simulink model "circuitElectrique"  (R2014b)
settings: Solver=ode23tb  StartTime=t0  StopTime=tf  MaxStep=max_step  MinStep=min_step  RelTol=tol
StopFcn:
  | save(wSaveFileName,wLinearOutputName,wNonLinearOutputName)
values from neighbouring files (symbols this model uses):
  A = [-3/(8*Ca)*Ei_mean^2-1/(R*Ca), 1/Ca;-1/L,0]    [circuitElectriqueDataDictionnary (Copie en conflit de Adam Burney 2015-02-07).m]    (also in circuitElectriqueDataDictionnary.m)
  Ai = Ais(i)    [circuitElectriqueDataDictionnary (Copie en conflit de Adam Burney 2015-02-07).m]    (also in circuitElectriqueDataDictionnary.m)
  alpha = 3    [circuitElectriqueDataDictionnary (Copie en conflit de Adam Burney 2015-02-07).m]    (also in circuitElectriqueDataDictionnary.m)
  B = [1/(R*Ca);1/L]    [circuitElectriqueDataDictionnary (Copie en conflit de Adam Burney 2015-02-07).m]    (also in circuitElectriqueDataDictionnary.m)
  C = eye(2)    [circuitElectriqueDataDictionnary (Copie en conflit de Adam Burney 2015-02-07).m]    (also in circuitElectriqueDataDictionnary.m)
  D = [0;0]    [circuitElectriqueDataDictionnary (Copie en conflit de Adam Burney 2015-02-07).m]    (also in circuitElectriqueDataDictionnary.m)
  Ei = 2    [circuitElectriqueDataDictionnary (Copie en conflit de Adam Burney 2015-02-07).m]    (also in circuitElectriqueDataDictionnary.m)
  Io = 1/8    (= 0.125)    [circuitElectriqueDataDictionnary (Copie en conflit de Adam Burney 2015-02-07).m]    (also in circuitElectriqueDataDictionnary.m)
  L = 3    [circuitElectriqueDataDictionnary (Copie en conflit de Adam Burney 2015-02-07).m]    (also in circuitElectriqueDataDictionnary.m)
  R = 1    [circuitElectriqueDataDictionnary (Copie en conflit de Adam Burney 2015-02-07).m]    (also in circuitElectriqueDataDictionnary.m)
  u0 = Ei_mean    (= 2)    [circuitElectriqueDataDictionnary (Copie en conflit de Adam Burney 2015-02-07).m]    (also in circuitElectriqueDataDictionnary.m)
  Vo = 1    [circuitElectriqueDataDictionnary (Copie en conflit de Adam Burney 2015-02-07).m]    (also in circuitElectriqueDataDictionnary.m)
  x0 = [Ei_mean;1/8*Ei_mean^3]    [circuitElectriqueDataDictionnary (Copie en conflit de Adam Burney 2015-02-07).m]    (also in circuitElectriqueDataDictionnary.m)
undefined symbols (not defined in the file or in its folder): pow
undefined symbols (not defined in the file): Ca
libraries: powerlib x10
settings Model: Creator=Zangdaarr  LastModifiedBy=Zangdaarr
settings DebuggingCC: MultiTaskDSMMsg=warning  MultiTaskCondExecSysMsg=none
settings RTWCC: IncludeERTFirstTime=on

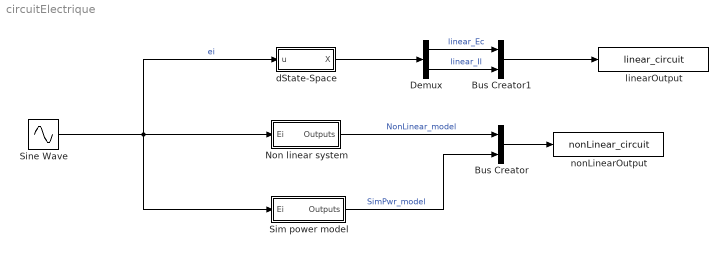
== system circuitElectrique ==
  Bus Creator : BusCreator  Inputs=2
  Bus Creator1 : BusCreator  Inputs=2
  Demux : Demux  Outputs=2
  Non linear system : Subsystem  mask{R=R, C=Ca, L=L, A=A, alpha=alpha}
  Sim power model : Subsystem  mask{Io=Io, Vo=Vo, alpha=alpha, R=R, C=Ca, L=L}
  Sine Wave : Sin  Amplitude=Ai  Bias=Ei  SampleTime=0
  dState-Space : Subsystem
  linearOutput : ToWorkspace  VariableName=linear_circuit  SaveFormat=Timeseries  SampleTime=-1
  nonLinearOutput : ToWorkspace  VariableName=nonLinear_circuit  SaveFormat=Timeseries  SampleTime=-1
  wires:
  Sine Wave/1 -> dState-Space/1(u), Sim power model/1(Ei), Non linear system/1(Ei)  "ei"
  Sim power model/1(Outputs) -> Bus Creator/2  "SimPwr_model"
  Non linear system/1(Outputs) -> Bus Creator/1  "NonLinear_model"
  Bus Creator/1 -> nonLinearOutput/1
  Demux/1 -> Bus Creator1/1  "linear_Ec"
  Demux/2 -> Bus Creator1/2  "linear_Il"
  Bus Creator1/1 -> linearOutput/1
  dState-Space/1(X) -> Demux/1

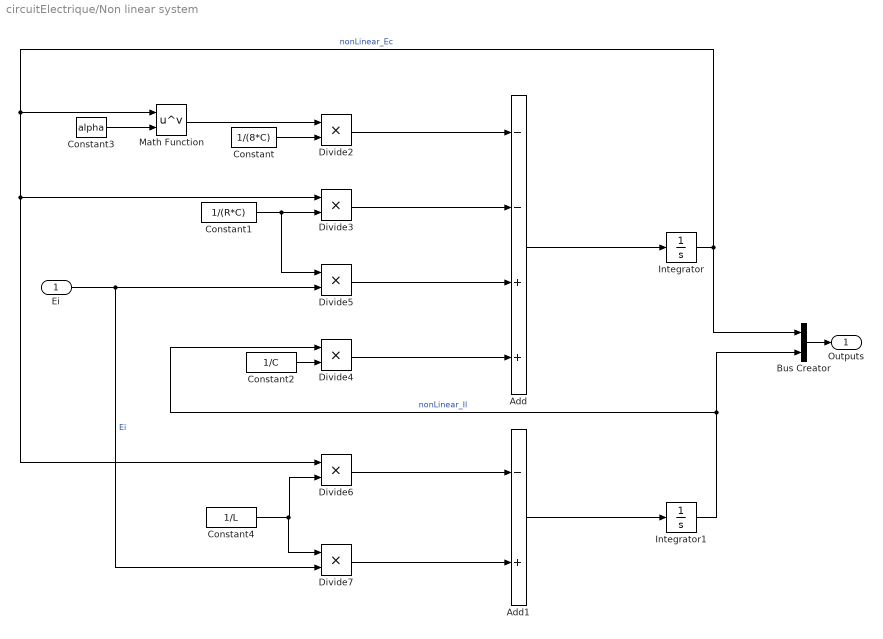
== system circuitElectrique/Non linear system ==
  Ei : Inport
  Add : Sum  Inputs=--++
  Add1 : Sum  Inputs=-+
  Bus Creator : BusCreator  Inputs=2
  Constant : Constant  Value=1/(8*C)
  Constant1 : Constant  Value=1/(R*C)
  Constant2 : Constant  Value=1/C
  Constant3 : Constant  Value=alpha
  Constant4 : Constant  Value=1/L
  Divide{2..7} (6 alike) : Product  Inputs=**
  Integrator : Integrator
  Integrator1 : Integrator
  Math Function : Math  Operator=pow  SaturateOnIntegerOverflow=on
  Outputs : Outport
  wires:
  Math Function/1 -> Divide2/1
  Constant/1 -> Divide2/2
  Constant1/1 -> Divide5/1, Divide3/2
  Constant2/1 -> Divide4/2
  Integrator1/1 -> Divide4/1, Bus Creator/2  "nonLinear_Il"
  Ei/1 -> Divide7/2, Divide5/2  "Ei"
  Divide2/1 -> Add/1
  Divide3/1 -> Add/2
  Divide5/1 -> Add/3
  Divide4/1 -> Add/4
  Add/1 -> Integrator/1
  Integrator/1 -> Bus Creator/1, Divide6/1, Divide3/1, Math Function/1  "nonLinear_Ec"
  Constant4/1 -> Divide7/1, Divide6/2
  Divide6/1 -> Add1/1
  Divide7/1 -> Add1/2
  Add1/1 -> Integrator1/1
  Bus Creator/1 -> Outputs/1
  Constant3/1 -> Math Function/2

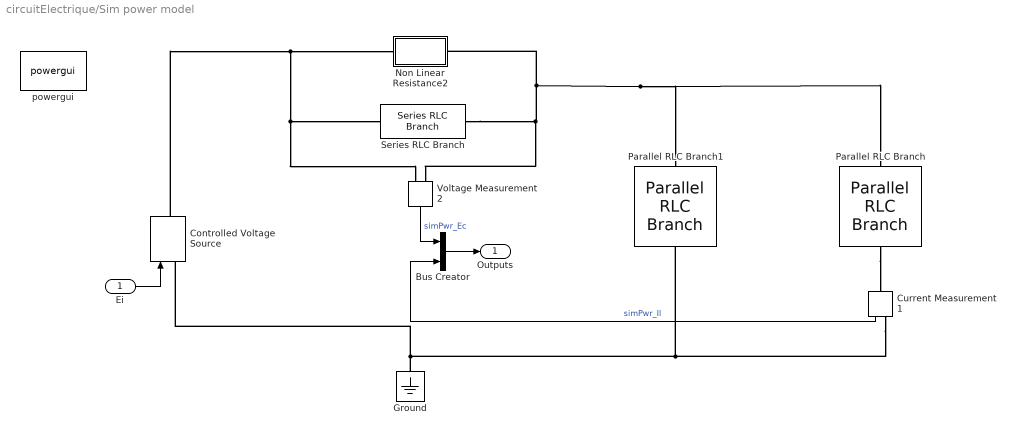
== system circuitElectrique/Sim power model ==
  Ei : Inport
  Bus Creator : BusCreator  Inputs=2
  Controlled Voltage Source : powerlib/Electrical Sources/Controlled Voltage Source  Initialize=on  Source_Type=AC  Amplitude=10  Phase=0  Frequency=0  Measurements=None
  Current Measurement1 : powerlib/Measurements/Current Measurement  PhasorSimulation=off  OutputType=Complex  PSBequivalent=0
  Ground : powerlib/Elements/Ground  LConnTagsString=a
  Non Linear Resistance2 : Subsystem  mask{Io=Io, Vo=Vo, alpha=alpha}
      mask prompts: alpha "a"
  Parallel RLC Branch : powerlib/Elements/Parallel RLC Branch  LConnTagsString=a  RConnTagsString=__new0  BranchType=L  Resistance=R  Inductance=L  SetiL0=on  InitialCurrent=0  Capacitance=1e-6  Setx0=off  InitialVoltage=0  Measurements=Branch current
  Parallel RLC Branch1 : powerlib/Elements/Parallel RLC Branch  LConnTagsString=a  RConnTagsString=__new0  BranchType=R  Resistance=R  Inductance=L  SetiL0=on  InitialCurrent=0  Capacitance=1e-6  Setx0=off  InitialVoltage=0  Measurements=Branch current
  Series RLC Branch : powerlib/Elements/Series RLC Branch  LConnTagsString=__new0  RConnTagsString=__new0  BranchType=C  Resistance=1  Inductance=1e-3  SetiL0=off  InitialCurrent=0  Capacitance=C  Setx0=on  InitialVoltage=0  Measurements=None
  Voltage Measurement2 : powerlib/Measurements/Voltage Measurement  PhasorSimulation=off  OutputType=Complex  PSBequivalent=0
  powergui : powerlib/powergui  Priority=1  SimulationMode=Continuous  SolverType=Tustin  SampleTime=100  frequency=60  SPID=off  DisableSnubberDevices=off  DisableRonSwitches=off  DisableVfSwitches=off  SwTol=0  DisplayEquations=off  Interpol=off  methode=off  Ts=0  frequencyindice=0  Pbase=100e6  ErrMax=1e-4  Iterations=50  UnitsV=kV  UnitsW=MW  FunctionMessages=off  echomessages=off  HookPort=off  EnableUseOfTLC=off  x0status=blocks  RestoreLinks=warning  ResistiveCurrentMeasurement=off  Frange=[0:2:500]  Ylog=off  Xlog=on  ShowGrid=off  save=off  variable=ZData  structure=0  ZoomFFT=off  StartTime=0.0  cycles=1  DisplayStyle=1  fundamental=60  FreqAxis=off  MaxFrequency=1000  frequencyindicesteady=1  RmsSteady=1  display=off
  Outputs : Outport
  wires:
  Voltage Measurement2/1 -> Bus Creator/1  "simPwr_Ec"
  Current Measurement1/1 -> Bus Creator/2  "simPwr_Il"
  Bus Creator/1 -> Outputs/1
  Ei/1 -> Controlled Voltage Source/1
  connections:
  Controlled Voltage Source/RConn1 -- Non Linear Resistance2/LConn1 -- Series RLC Branch/LConn1 -- Voltage Measurement2/LConn1
  Parallel RLC Branch/RConn1 -- Current Measurement1/LConn1
  Series RLC Branch/RConn1 -- Voltage Measurement2/LConn2 -- Non Linear Resistance2/RConn1 -- Parallel RLC Branch/LConn1 -- Parallel RLC Branch1/LConn1
  Current Measurement1/RConn1 -- Parallel RLC Branch1/RConn1 -- Controlled Voltage Source/LConn1 -- Ground/LConn1

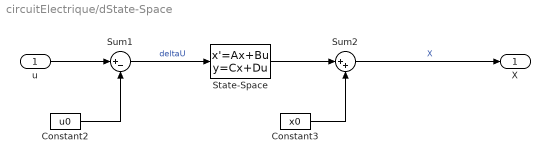
== system circuitElectrique/dState-Space ==
  u : Inport
  Constant2 : Constant  Value=u0
  Constant3 : Constant  Value=x0
  State-Space : StateSpace  A=A  B=B  C=C  D=D  X0=0
  Sum1 : Sum  Inputs=|+-
  Sum2 : Sum  Inputs=|++
  X : Outport
  wires:
  u/1 -> Sum1/1
  Constant3/1 -> Sum2/2
  Sum2/1 -> X/1  "X"
  Constant2/1 -> Sum1/2
  Sum1/1 -> State-Space/1  "deltaU"
  State-Space/1 -> Sum2/1

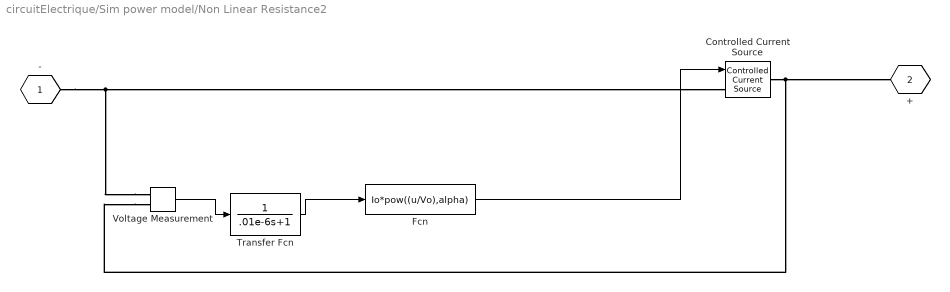
== system circuitElectrique/Sim power model/Non Linear Resistance2 ==
  Controlled Current Source : powerlib/Electrical Sources/Controlled Current Source  Initialize=on  Source_Type=AC  Amplitude=0  Phase=0  Frequency=0  Measurements=Current
  Fcn : Fcn  Expr=Io*pow((u/Vo),alpha)
  Transfer Fcn : TransferFcn  Denominator=[.01e-6 1]
  Voltage Measurement : powerlib/Measurements/Voltage Measurement  PhasorSimulation=off  OutputType=Complex  PSBequivalent=0
  - : PMIOPort  Tag=PMCPort  Port=1  Side=Left
  + : PMIOPort  Tag=PMCPort  Port=2  Side=Right
  wires:
  Transfer Fcn/1 -> Fcn/1
  Fcn/1 -> Controlled Current Source/1
  Voltage Measurement/1 -> Transfer Fcn/1
  connections:
  Voltage Measurement/LConn2 -- +/RConn1 -- Controlled Current Source/RConn1
  Voltage Measurement/LConn1 -- Controlled Current Source/LConn1 -- -/RConn1
